simulink model "flight_model"  (Simulink 7.6)
settings: Solver=ode23  StartTime=0.0  StopTime=30  RelTol=1e-3
values from neighbouring files (symbols this model uses):
  initial_pos = [[44.98 -76.96] * pi / 180 0]    [Geo_model_sim.m]
  Uo = trim_values(10:13)    [Geo_Find_Trim.m]
  Xo = trim_values(1:9)    [Geo_Find_Trim.m]
undefined symbols (not defined in the file or in its folder): aerosimlib, Earth, WGS
settings Model: Creator=gblouin  LastModifiedBy=aholtzma
settings DataIOCC: ExternalInput=[u]  LimitDataPoints=off  SaveOutput=off  SignalLogging=off  DSMLogging=off  OutputSaveName=xout
settings OptimizationCC: InlineParams=on  InlineInvariantSignals=on  EfficientFloat2IntCast=on
settings DebuggingCC: SaveWithParameterizedLinksMsg=none  MultiTaskDSMMsg=warning  MultiTaskCondExecSysMsg=none  StrictBusMsg=Warning
settings SFSimCC: SimParseCustomCode=off
settings RTWCC: IncludeERTFirstTime=on
settings GRTTargetCC: TargetFcnLib=ansi_tfl_tmw.mat

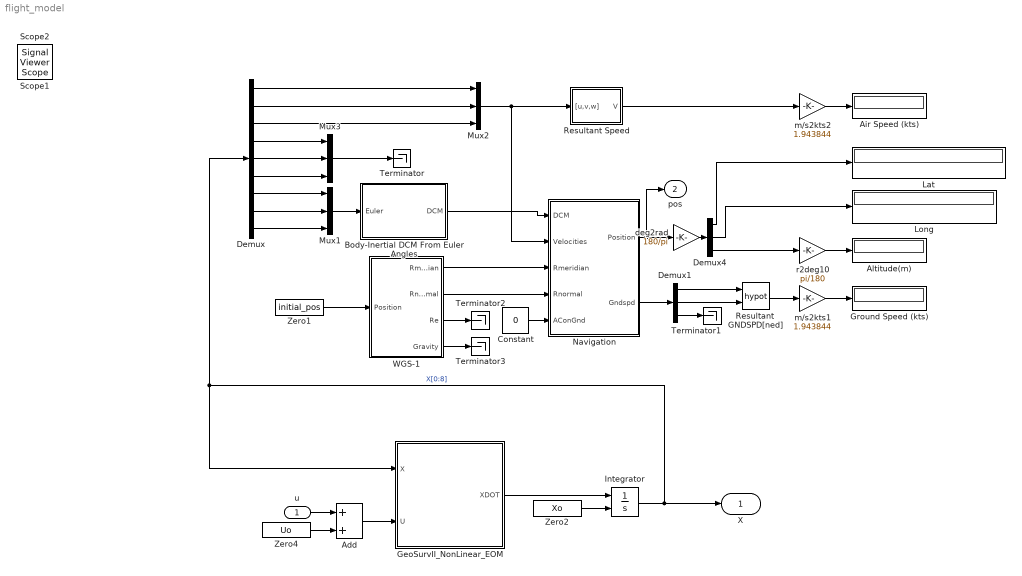
== system flight_model ==
  u : Inport  PortDimensions=4
  Add : Sum
  Air Speed (kts) : Display
  Altitude(m) : Display
  Body-Inertial DCM From Euler Angles : Subsystem  AncestorBlock=aerosimlib/Transformations/Body-Inertial DCM From Euler Angles
  Constant : Constant  Value=0
  Demux : Demux  Outputs=9
  Demux1 : Demux  Outputs=3
  Demux4 : Demux  Outputs=3
  GeoSurvII_NonLinear_EOM : Stateflow chart  TreatAsAtomicUnit=on
  Ground Speed (kts) : Display
  Integrator : Integrator  InitialConditionSource=external  InitialCondition=Xo
  Lat : Display
  Long : Display
  Mux1 : Mux  Inputs=3
  Mux2 : Mux  Inputs=3
  Mux3 : Mux  Inputs=3
  Navigation : Subsystem
  Resultant  GNDSPD[ned] : Math  Operator=hypot  SaturateOnIntegerOverflow=on
  Resultant Speed : Subsystem  AncestorBlock=aerosimlib/Equations of Motion/Body-Frame EOM/Kinematics (Euler)
  Terminator{,1..3} (4 alike) : Terminator
  WGS-1 : Subsystem  AncestorBlock=aerosimlib/Earth/WGS-84
  Zero1 : Constant  Value=initial_pos
  Zero2 : Constant  Value=Xo
  Zero4 : Constant  Value=Uo
  deg2rad : Gain  Gain=180/pi
  m/s2kts1 : Gain  Gain=1.943844
  m/s2kts2 : Gain  Gain=1.943844
  r2deg10 : Gain  Gain=pi/180
  X : Outport
  pos : Outport  Port=2
  Scope1 : SignalViewerScope  IOType=viewer  NumInputPorts=2  ZoomMode=xonly  RefreshTime=1.500000
      settings: TimeRange=100  YMin=-3.5~-2.84987e-012  YMax=0.5~-2.57845e-012  MaxDataPoints=20000
  Scope2 : SignalViewerScope  IOType=viewer  NumInputPorts=2  ZoomMode=xonly  RefreshTime=1.500000
      settings: TimeRange=100  YMin=-40~9.16954  YMax=10~10.1348  MaxDataPoints=20000
  wires:
  Navigation/1(Position) -> deg2rad/1, pos/1
  Demux4/1 -> Lat/1
  Demux4/2 -> Long/1
  deg2rad/1 -> Demux4/1
  Demux4/3 -> r2deg10/1
  r2deg10/1 -> Altitude(m)/1
  Navigation/2(Gndspd) -> Demux1/1
  Demux1/1 -> Resultant  GNDSPD[ned]/1
  Demux1/2 -> Resultant  GNDSPD[ned]/2
  Integrator/1 -> GeoSurvII_NonLinear_EOM/1(X), Demux/1, X/1  "X[0:8]"
  Zero2/1 -> Integrator/2
  GeoSurvII_NonLinear_EOM/1(XDOT) -> Integrator/1
  Demux/1 -> Mux2/1
  Resultant  GNDSPD[ned]/1 -> m/s2kts1/1
  m/s2kts1/1 -> Ground Speed (kts)/1
  WGS-1/1(Rmeridian) -> Navigation/3(Rmeridian)
  WGS-1/2(Rnormal) -> Navigation/4(Rnormal)
  Body-Inertial DCM From Euler Angles/1(DCM) -> Navigation/1(DCM)
  Mux2/1 -> Navigation/2(Velocities), Resultant Speed/1("[u,v,w]")
  Zero1/1 -> WGS-1/1(Position)
  Resultant Speed/1(V) -> m/s2kts2/1
  m/s2kts2/1 -> Air Speed (kts)/1
  Demux/2 -> Mux2/2
  Demux/3 -> Mux2/3
  Demux/7 -> Mux1/1
  Demux/8 -> Mux1/2
  Demux/9 -> Mux1/3
  Mux1/1 -> Body-Inertial DCM From Euler Angles/1(Euler)
  Demux/4 -> Mux3/1
  Demux/5 -> Mux3/2
  Demux/6 -> Mux3/3
  Add/1 -> GeoSurvII_NonLinear_EOM/2(U)
  u/1 -> Add/1
  Zero4/1 -> Add/2
  Mux3/1 -> Terminator/1
  Demux1/3 -> Terminator1/1
  WGS-1/3(Re) -> Terminator2/1
  WGS-1/4(Gravity) -> Terminator3/1
  Constant/1 -> Navigation/5(AConGnd)

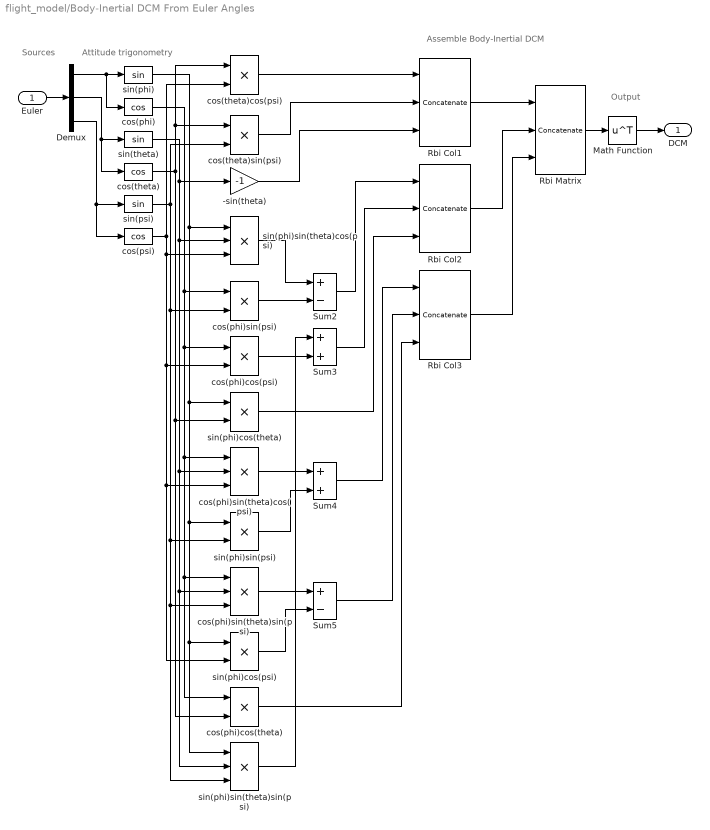
== system flight_model/Body-Inertial DCM From Euler Angles ==
  note: Sources
  note: Assemble Body-Inertial DCM
  note: Output
  note: Attitude trigonometry
  Euler : Inport  PortDimensions=[3 1]
  -sin(theta) : Gain  Gain=-1  SaturateOnIntegerOverflow=on  OutDataTypeStr=Inherit: Same as input  ParamDataTypeStr=Inherit: Same as input
  Demux : Demux  Outputs=3
  Math Function : Math  Operator=transpose  SaturateOnIntegerOverflow=on
  Rbi Matrix : Concatenate  NumInputs=3  Mode=Multidimensional array  ConcatenateDimension=2
  Rbi Col1 : Concatenate  NumInputs=3  Mode=Multidimensional array
  Rbi Col2 : Concatenate  NumInputs=3  Mode=Multidimensional array
  Rbi Col3 : Concatenate  NumInputs=3  Mode=Multidimensional array
  Sum2 : Sum  Inputs=+-  SaturateOnIntegerOverflow=on  InputSameDT=on  OutDataTypeStr=Inherit: Same as first input
  Sum3 : Sum  SaturateOnIntegerOverflow=on  InputSameDT=on  OutDataTypeStr=Inherit: Same as first input
  Sum4 : Sum  SaturateOnIntegerOverflow=on  InputSameDT=on  OutDataTypeStr=Inherit: Same as first input
  Sum5 : Sum  Inputs=+-  SaturateOnIntegerOverflow=on  InputSameDT=on  OutDataTypeStr=Inherit: Same as first input
  cos(phi) : Trigonometry  Operator=cos
  cos(phi)cos(psi) : Product  SaturateOnIntegerOverflow=on  InputSameDT=on  OutDataTypeStr=Inherit: Same as first input
  cos(phi)cos(theta) : Product  SaturateOnIntegerOverflow=on  InputSameDT=on  OutDataTypeStr=Inherit: Same as first input
  cos(phi)sin(psi) : Product  SaturateOnIntegerOverflow=on  InputSameDT=on  OutDataTypeStr=Inherit: Same as first input
  cos(phi)sin(theta)cos(psi) : Product  Inputs=3  SaturateOnIntegerOverflow=on  InputSameDT=on  OutDataTypeStr=Inherit: Same as first input
  cos(phi)sin(theta)sin(psi) : Product  Inputs=3  SaturateOnIntegerOverflow=on  InputSameDT=on  OutDataTypeStr=Inherit: Same as first input
  cos(psi) : Trigonometry  Operator=cos
  cos(theta) : Trigonometry  Operator=cos
  cos(theta)cos(psi) : Product  SaturateOnIntegerOverflow=on  InputSameDT=on  OutDataTypeStr=Inherit: Same as first input
  cos(theta)sin(psi) : Product  SaturateOnIntegerOverflow=on  InputSameDT=on  OutDataTypeStr=Inherit: Same as first input
  sin(phi) : Trigonometry
  sin(phi)cos(psi) : Product  SaturateOnIntegerOverflow=on  InputSameDT=on  OutDataTypeStr=Inherit: Same as first input
  sin(phi)cos(theta) : Product  SaturateOnIntegerOverflow=on  InputSameDT=on  OutDataTypeStr=Inherit: Same as first input
  sin(phi)sin(psi) : Product  SaturateOnIntegerOverflow=on  InputSameDT=on  OutDataTypeStr=Inherit: Same as first input
  sin(phi)sin(theta)cos(psi) : Product  Inputs=3  SaturateOnIntegerOverflow=on  InputSameDT=on  OutDataTypeStr=Inherit: Same as first input
  sin(phi)sin(theta)sin(psi) : Product  Inputs=3  SaturateOnIntegerOverflow=on  InputSameDT=on  OutDataTypeStr=Inherit: Same as first input
  sin(psi) : Trigonometry
  sin(theta) : Trigonometry
  DCM : Outport
  wires:
  Euler/1 -> Demux/1
  Rbi Col1/1 -> Rbi Matrix/1
  Rbi Col2/1 -> Rbi Matrix/2
  Rbi Col3/1 -> Rbi Matrix/3
  Rbi Matrix/1 -> Math Function/1
  Demux/1 -> sin(phi)/1, cos(phi)/1
  Demux/2 -> cos(theta)/1, sin(theta)/1
  Demux/3 -> cos(psi)/1, sin(psi)/1
  sin(phi)/1 -> sin(phi)sin(psi)/1, sin(phi)cos(psi)/1, sin(phi)sin(theta)sin(psi)/1, sin(phi)cos(theta)/1, sin(phi)sin(theta)cos(psi)/1
  cos(phi)/1 -> cos(phi)cos(theta)/1, cos(phi)sin(theta)sin(psi)/1, cos(phi)sin(theta)cos(psi)/1, cos(phi)cos(psi)/1, cos(phi)sin(psi)/1
  sin(theta)/1 -> cos(phi)sin(theta)cos(psi)/2, cos(phi)sin(theta)sin(psi)/2, sin(phi)sin(theta)sin(psi)/2, sin(phi)sin(theta)cos(psi)/2, -sin(theta)/1
  cos(theta)/1 -> cos(phi)cos(theta)/2, sin(phi)cos(theta)/2, cos(theta)sin(psi)/1, cos(theta)cos(psi)/1
  sin(psi)/1 -> sin(phi)sin(psi)/2, cos(phi)sin(theta)sin(psi)/3, sin(phi)sin(theta)sin(psi)/3, cos(phi)sin(psi)/2, cos(theta)sin(psi)/2
  cos(psi)/1 -> sin(phi)cos(psi)/2, cos(phi)sin(theta)cos(psi)/3, cos(phi)cos(psi)/2, sin(phi)sin(theta)cos(psi)/3, cos(theta)cos(psi)/2
  cos(phi)sin(psi)/1 -> Sum2/2
  cos(phi)cos(psi)/1 -> Sum3/2
  sin(phi)sin(theta)cos(psi)/1 -> Sum2/1
  cos(phi)sin(theta)cos(psi)/1 -> Sum4/1
  sin(phi)sin(psi)/1 -> Sum4/2
  cos(phi)sin(theta)sin(psi)/1 -> Sum5/1
  sin(phi)cos(psi)/1 -> Sum5/2
  cos(theta)cos(psi)/1 -> Rbi Col1/1
  cos(theta)sin(psi)/1 -> Rbi Col1/2
  -sin(theta)/1 -> Rbi Col1/3
  Sum2/1 -> Rbi Col2/1
  Sum3/1 -> Rbi Col2/2
  sin(phi)cos(theta)/1 -> Rbi Col2/3
  Sum4/1 -> Rbi Col3/1
  Sum5/1 -> Rbi Col3/2
  cos(phi)cos(theta)/1 -> Rbi Col3/3
  Math Function/1 -> DCM/1
  sin(phi)sin(theta)sin(psi)/1 -> Sum3/1

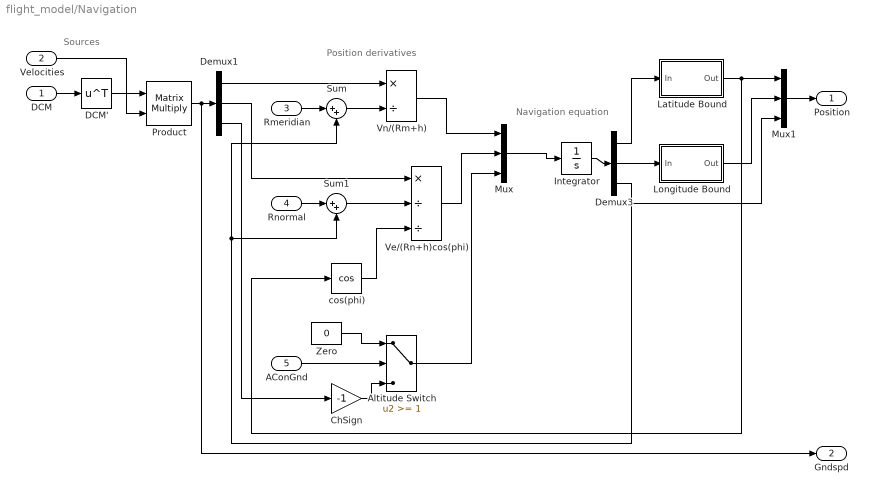
== system flight_model/Navigation ==
  note: Navigation equation
  note: Position derivatives
  note: Sources
  DCM : Inport  PortDimensions=[3 3]
  Velocities : Inport  Port=2  PortDimensions=[3 1]
  Rmeridian : Inport  Port=3  PortDimensions=1
  Rnormal : Inport  Port=4  PortDimensions=1
  AConGnd : Inport  Port=5  PortDimensions=1
  Altitude Switch : Switch  Threshold=1  SaturateOnIntegerOverflow=on  InputSameDT=on
  ChSign : Gain  Gain=-1  SaturateOnIntegerOverflow=on  OutDataTypeStr=Inherit: Same as input  ParamDataTypeStr=Inherit: Same as input
  DCM' : Math  Operator=transpose  SaturateOnIntegerOverflow=on
  Demux1 : Demux  Outputs=3
  Demux3 : Demux  Outputs=3
  Integrator : Integrator  InitialCondition=[41.684028*pi/180 -81.389750*pi/180 500]
  Latitude Bound : Subsystem
      mask Type: Latitude bound
      mask Description: Bounds the latitude to [-pi/2, pi/2]. When the lower bound is exceeded the latitude is increasing again; when the upper bound is exceeded the latitude is decreasing.
  Longitude Bound : Subsystem
      mask Type: Longitude bound
      mask Description: Bounds the longitude to [-pi, pi]. When -pi bound is exceeded the longitude wraps back to pi; when the pi bound is exceeded the longitude wraps back to -pi.
  Mux : Mux  Inputs=3
  Mux1 : Mux  Inputs=3
  Product : Product  Multiplication=Matrix(*)  SaturateOnIntegerOverflow=on  InputSameDT=on  OutDataTypeStr=Inherit: Same as first input
  Sum : Sum  Inputs=|++  SaturateOnIntegerOverflow=on  InputSameDT=on  OutDataTypeStr=Inherit: Same as first input
  Sum1 : Sum  Inputs=|++  SaturateOnIntegerOverflow=on  InputSameDT=on  OutDataTypeStr=Inherit: Same as first input
  Ve/(Rn+h)cos(phi) : Product  Inputs=*//  SaturateOnIntegerOverflow=on  InputSameDT=on  OutDataTypeStr=Inherit: Same as first input
  Vn/(Rm+h) : Product  Inputs=*/  SaturateOnIntegerOverflow=on  InputSameDT=on  OutDataTypeStr=Inherit: Same as first input
  Zero : Constant  Value=0
  cos(phi) : Trigonometry  Operator=cos
  Position : Outport
  Gndspd : Outport  Port=2
  wires:
  Latitude Bound/1(Out) -> Mux1/1, cos(phi)/1
  Mux1/1 -> Position/1
  Longitude Bound/1(Out) -> Mux1/2
  Demux3/1 -> Latitude Bound/1(In)
  Demux3/2 -> Longitude Bound/1(In)
  Demux3/3 -> Mux1/3, Sum1/2, Sum/2
  cos(phi)/1 -> Ve/(Rn+h)cos(phi)/3
  Integrator/1 -> Demux3/1
  Mux/1 -> Integrator/1
  Altitude Switch/1 -> Mux/3
  ChSign/1 -> Altitude Switch/3
  Zero/1 -> Altitude Switch/1
  AConGnd/1 -> Altitude Switch/2
  DCM'/1 -> Product/1
  DCM/1 -> DCM'/1
  Ve/(Rn+h)cos(phi)/1 -> Mux/2
  Sum1/1 -> Ve/(Rn+h)cos(phi)/2
  Vn/(Rm+h)/1 -> Mux/1
  Sum/1 -> Vn/(Rm+h)/2
  Rnormal/1 -> Sum1/1
  Rmeridian/1 -> Sum/1
  Product/1 -> Gndspd/1, Demux1/1
  Demux1/2 -> Ve/(Rn+h)cos(phi)/1
  Demux1/3 -> ChSign/1
  Demux1/1 -> Vn/(Rm+h)/1
  Velocities/1 -> Product/2

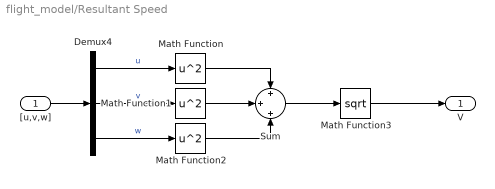
== system flight_model/Resultant Speed ==
  "[u,v,w]" : Inport  PortDimensions=[3 1]
  Demux4 : Demux  Outputs=3
  Math Function : Math  Operator=square  SaturateOnIntegerOverflow=on
  Math Function1 : Math  Operator=square  SaturateOnIntegerOverflow=on
  Math Function2 : Math  Operator=square  SaturateOnIntegerOverflow=on
  Math Function3 : Math  Operator=sqrt  SaturateOnIntegerOverflow=on
  Sum : Sum  Inputs=+|+|+
  V : Outport
  wires:
  Demux4/2 -> Math Function1/1  "v"
  Demux4/3 -> Math Function2/1  "w"
  Math Function/1 -> Sum/1
  Math Function1/1 -> Sum/2
  Math Function2/1 -> Sum/3
  Sum/1 -> Math Function3/1
  Math Function3/1 -> V/1
  Demux4/1 -> Math Function/1  "u"
  "[u,v,w]"/1 -> Demux4/1

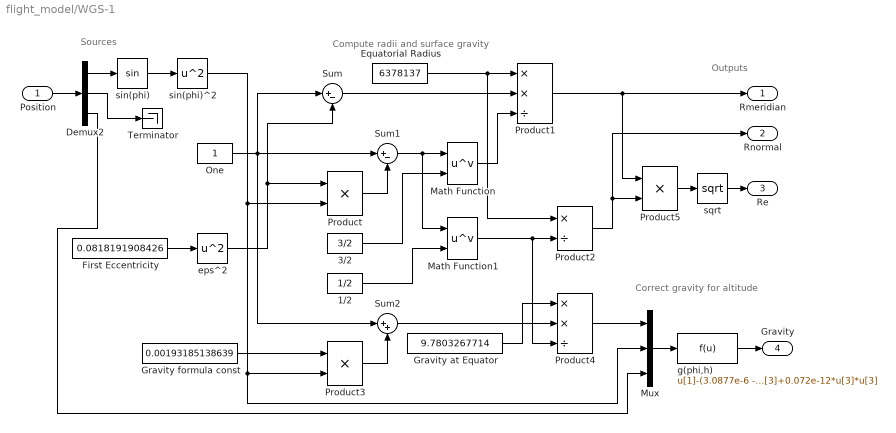
== system flight_model/WGS-1 ==
  note: Sources
  note: Compute radii and surface gravity
  note: Correct gravity for altitude
  note: Outputs
  Position : Inport
  1/2 : Constant  Value=1/2
  3/2 : Constant  Value=3/2
  Demux2 : Demux  Outputs=3
  Equatorial Radius : Constant  Value=6378137
  First Eccentricity : Constant  Value=0.0818191908426
  Gravity at Equator : Constant  Value=9.7803267714
  Gravity formula const : Constant  Value=0.00193185138639
  Math Function : Math  Operator=pow  SaturateOnIntegerOverflow=on
  Math Function1 : Math  Operator=pow  SaturateOnIntegerOverflow=on
  Mux : Mux  Inputs=3
  One : Constant
  Product : Product  SaturateOnIntegerOverflow=on  InputSameDT=on  OutDataTypeStr=Inherit: Same as first input
  Product1 : Product  Inputs=**/  SaturateOnIntegerOverflow=on  InputSameDT=on  OutDataTypeStr=Inherit: Same as first input
  Product2 : Product  Inputs=*/  SaturateOnIntegerOverflow=on  InputSameDT=on  OutDataTypeStr=Inherit: Same as first input
  Product3 : Product  SaturateOnIntegerOverflow=on  InputSameDT=on  OutDataTypeStr=Inherit: Same as first input
  Product4 : Product  Inputs=**/  SaturateOnIntegerOverflow=on  InputSameDT=on  OutDataTypeStr=Inherit: Same as first input
  Product5 : Product  SaturateOnIntegerOverflow=on  InputSameDT=on  OutDataTypeStr=Inherit: Same as first input
  Sum : Sum  Inputs=|+-  SaturateOnIntegerOverflow=on  InputSameDT=on  OutDataTypeStr=Inherit: Same as first input
  Sum1 : Sum  Inputs=|+-  SaturateOnIntegerOverflow=on  InputSameDT=on  OutDataTypeStr=Inherit: Same as first input
  Sum2 : Sum  Inputs=|++  SaturateOnIntegerOverflow=on  InputSameDT=on  OutDataTypeStr=Inherit: Same as first input
  Terminator : Terminator
  eps^2 : Math  Operator=square  SaturateOnIntegerOverflow=on
  g(phi,h) : Fcn  Expr=u[1]-(3.0877e-6 - 0.0044e-6*u[2])*u[3]+0.072e-12*u[3]*u[3]
  sin(phi) : Trigonometry
  sin(phi)^2 : Math  Operator=square  SaturateOnIntegerOverflow=on
  sqrt : Math  Operator=sqrt  SaturateOnIntegerOverflow=on
  Rmeridian : Outport
  Rnormal : Outport  Port=2
  Re : Outport  Port=3
  Gravity : Outport  Port=4
  wires:
  sqrt/1 -> Re/1
  Product5/1 -> sqrt/1
  First Eccentricity/1 -> eps^2/1
  eps^2/1 -> Sum/2, Product/1
  sin(phi)/1 -> sin(phi)^2/1
  sin(phi)^2/1 -> Product/2, Product3/2, Mux/2
  One/1 -> Sum1/1, Sum2/1, Sum/1
  Product/1 -> Sum1/2
  Sum1/1 -> Math Function/1, Math Function1/1
  3/2/1 -> Math Function/2
  1/2/1 -> Math Function1/2
  Equatorial Radius/1 -> Product1/1, Product2/1
  Sum/1 -> Product1/2
  Math Function/1 -> Product1/3
  Math Function1/1 -> Product2/2, Product4/3
  Product1/1 -> Rmeridian/1, Product5/1
  Product2/1 -> Rnormal/1, Product5/2
  Gravity formula const/1 -> Product3/1
  Product3/1 -> Sum2/2
  Gravity at Equator/1 -> Product4/1
  Sum2/1 -> Product4/2
  Product4/1 -> Mux/1
  Position/1 -> Demux2/1
  Demux2/1 -> sin(phi)/1
  Demux2/2 -> Terminator/1
  Mux/1 -> g(phi,h)/1
  g(phi,h)/1 -> Gravity/1
  Demux2/3 -> Mux/3

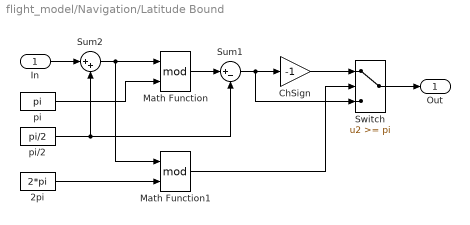
== system flight_model/Navigation/Latitude Bound ==
  In : Inport
  2pi : Constant  Value=2*pi
  ChSign : Gain  Gain=-1  SaturateOnIntegerOverflow=on  OutDataTypeStr=Inherit: Same as input  ParamDataTypeStr=Inherit: Same as input
  Math Function : Math  Operator=mod  SaturateOnIntegerOverflow=on
  Math Function1 : Math  Operator=mod  SaturateOnIntegerOverflow=on
  Sum1 : Sum  Inputs=|+-  SaturateOnIntegerOverflow=on  InputSameDT=on  OutDataTypeStr=Inherit: Same as first input
  Sum2 : Sum  Inputs=|++  SaturateOnIntegerOverflow=on  InputSameDT=on  OutDataTypeStr=Inherit: Same as first input
  Switch : Switch  Threshold=pi  SaturateOnIntegerOverflow=on  InputSameDT=on
  pi : Constant  Value=pi
  pi/2 : Constant  Value=pi/2
  Out : Outport
  wires:
  2pi/1 -> Math Function1/2
  ChSign/1 -> Switch/1
  Sum2/1 -> Math Function1/1, Math Function/1
  In/1 -> Sum2/1
  Switch/1 -> Out/1
  Math Function1/1 -> Switch/2
  Sum1/1 -> Switch/3, ChSign/1
  pi/2/1 -> Sum2/2, Sum1/2
  Math Function/1 -> Sum1/1
  pi/1 -> Math Function/2

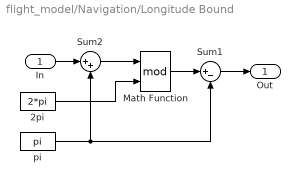
== system flight_model/Navigation/Longitude Bound ==
  In : Inport
  2pi : Constant  Value=2*pi
  Math Function : Math  Operator=mod  SaturateOnIntegerOverflow=on
  Sum1 : Sum  Inputs=|+-  SaturateOnIntegerOverflow=on  InputSameDT=on  OutDataTypeStr=Inherit: Same as first input
  Sum2 : Sum  Inputs=|++  SaturateOnIntegerOverflow=on  InputSameDT=on  OutDataTypeStr=Inherit: Same as first input
  pi : Constant  Value=pi
  Out : Outport
  wires:
  Math Function/1 -> Sum1/1
  2pi/1 -> Math Function/2
  In/1 -> Sum2/1
  Sum2/1 -> Math Function/1
  pi/1 -> Sum2/2, Sum1/2
  Sum1/1 -> Out/1

== matlab function GeoSurvII_NonLinear_EOM ==
  settings: fimath=|
      | fimath(...
      | 'RoundMode', 'floor',...
      | 'OverflowMode', 'wrap',...
      | 'ProductMode', 'KeepLSB', 'ProductWordLength', 32,...
      | 'SumMode', 'KeepLSB', 'SumWordLength', 32,...
      | 'CastBeforeSum', false)
  data: X input double; XDOT output double; U input double
function XDOT = Geo_model(X,U)

%GEO_MODEL Full 6 DOF model for GeoSurv II aircraft
%
%   [XDOT] = GEO_MODEL(X,U) returns the state derivatives, XDOT, given the
%   current state and inputs, X and U.  The constants are the nominal
%   constants.
%
%   State vector X and input vector U is defined as
%   
%       X = [u;v;w;p;q;r;phi;theta;psi] = [x1;x2;x3;x4;x5;x6;x7;x8;x9]
%       U = [d_A;d_E;d_R;d_th] = [u1;u2;u3;u4]
%
%
%Created by Christopher Lum
%lum@u.washington.edu
%Modified for GeoSurv II aircraft by Guillaume Blouin


%-----------------------CONSTANTS-------------------------------
%Unit conversions
lb_to_kg = 0.45359237;          %Unit conversion (pounds to kilograms)
in_to_m = 0.0254;               %Unit conversion (inches to meters)
ft_to_m = 0.3048;               %Unit conversion (feet to meters)
kt_to_ms = 0.514444;            %Unit conversion (knots to meters/second)
slug_to_kg = 14.593903;         %Unit conversion (slugs to kilograms)

%Mass moments of inertia
Ixx = 25.2589*slug_to_kg*ft_to_m^2;
Iyy = 32.8379*slug_to_kg*ft_to_m^2;
Izz = 47.0740*slug_to_kg*ft_to_m^2;
Ixz = 0*slug_to_kg*ft_to_m^2;

%Nominal vehicle constants (problem 1)
m = 186*lb_to_kg;               %Aircraft total mass (kg)
cbar = 27*in_to_m;              %Mean Aerodynamic Chord (m)
lt = 108.55*in_to_m;            %Distance by AC of tail and body (m)
S = 36*ft_to_m^2;               %Wing planform area (m^2)
St = 9.5*ft_to_m^2;             %Tail planform area (m^2)
i = -2*pi/180;                  %Tail incidence angle (rad)
AR = 7.11;                      %Aspect ratio
e = 0.836;                      %Oswalt's efficiency factor

Xcg = 0.25*cbar;                %x position of CoG in Fm (m)
Ycg = 0;                        %y position of CoG in Fm (m)
Zcg = 0.037*cbar;               %z position of CoG in Fm (m)

%Engine inputs
Xapt = 0;                       %x position of engine force in Fm (m)
Yapt = 0;                       %y position of engine force in Fm (m)
Zapt = 0.1405;                  %z position of engine force in Fm (m)

%Other constants
rho = 1.225;                    %Air density (kg/m^3)
g = 9.81;                       %Gravitational acceleration (m/s^2)
depsda = 0.33;                  %Change in downwash w.r.t. alpha (rad/rad)
alpha_L0 = -4*pi/180;           %Zero lift angle of attack (rad)

%Stability Derivatives (output from Justin Koning's Linear Model)
CXu = -0.096;
CXa = 0.19042;
CXadot = 0;
CXq = 0;
CXde = 0;
 
CZu = -1.0381;
CZa = -5.9345;
CZadot = -1.1763;
CZq = -5.6462;
CZde = -0.15543;
 
Cmu = 0;
Cma = -0.6094;
Cmadot = -4.496;
Cmq = -14.9865;
Cmde = -0.5958;
 
CYb = -0.5291;
CYbdot = 0;
CYp = 0.029801;
CYr = 0.4479;
CYda = 0;
CYdr = 0.13127;
 
Clb = -0.033192;
Clp = -0.49901;
Clr = 0.14677;
Clda = 0.14359;
Cldr = 0.0035059;
 
Cnb = 0.20878;
Cnbdot = 0;
Cnp = -0.071083;
Cnr = -0.20574;
Cnda = -0.0051955;
Cndr = -0.070618;

%Convert CZ to CL
CLu = -CZu;
CLa = -CZa;
CLadot = -CZadot;
CLq = -CZq;
CLde = -CZde;

%Other Stability Derivatives (from AERO database)
CDo = 0.0222;
CMo = -0.1003;
CLa_t = 3.544;


%--------------------------STATE VECTOR----------------------------------
%Extract state vector
x1 = X(1);                              %u
x2 = X(2);                              %v
x3 = X(3);                              %w
x4 = X(4);                              %p
x5 = X(5);                              %q
x6 = X(6);                              %r
x7 = X(7);                              %phi
x8 = X(8);                              %theta
x9 = X(9);                              %psi

u1 = U(1);                              %d_A (aileron)
u2 = U(2);                              %d_E (elevator)
u3 = U(3);                              %d_R (rudder)
u4 = U(4);                              %d_th (throttle)


%---------------INTERMEDIATE VARIABLES------------------------
%Calculate airspeed
Va = sqrt(x1^2 + x2^2 + x3^2);

%Calculate alpha and beta
alpha = atan(x3/x1);
beta = asin(x2/Va);

%Calculate dynamic pressure
Q = 0.5*rho*Va^2;

%Also define the vectors wbe_b and V_b 
wbe_b = [x4;x5;x6];
V_b = [x1;x2;x3];


%---------------AERODYNAMIC FORCE COEFFICIENTS----------------
%Calculate the CL_wb
if Va<(35.6*kt_to_ms)
end

if alpha<= 17*pi*180
    CL_wb=CLa*(alpha-alpha_L0);
elseif alpha>17*pi*180
    CL_wb=-5*10^-5*alpha^4+0.0034*alpha^3-0.092*alpha^2+1.1374*alpha-4.2971;
else
    CL_wb=2.75;
end

%Calculate CL_t
epsilon = depsda*(alpha - alpha_L0);
alpha_t = alpha - epsilon + i + CLq*x5*lt/Va;
CL_t = CLa_t*alpha_t + CLde*u2;

%Total lift force
CL = CL_wb + CL_t*(St/S);

%Total drag force (neglecting tail)
CD = CDo + CL^2/(pi*AR*e);

%Calculate sideforce
CY = CYb*beta + CYdr*u3 + CYr*x6;


%--------------DIMENSIONAL AERODYNAMIC FORCES---------------------
%Calculate the actual dimensional forces.  These are in F_s (stability axis)
FA_s = [-CD*Q*S;
         CY*Q*S;
        -CL*Q*S];
    
%Rotate these forces to F_b (body axis)
C_bs = [cos(alpha) 0 -sin(alpha);
        0 1 0;
        sin(alpha) 0 cos(alpha)];
    
FA_b = C_bs*FA_s;


%-------------AERODYNAMIC MOMENT COEFFICIENTS---------------
%Calculate the moments in Fb.  Define eta, dCMdx and dCMdu
eta11 = Clb*beta;
eta21 = CMo - (CLa_t*(St*lt)/(S*cbar))*(alpha - epsilon);
eta31 = Cnb*beta;

eta = [eta11;
       eta21;
       eta31];

dCMdx = (cbar/Va)*[Clp 0 Clr;
                    0 (Cmq*(St*lt^2)/(S*cbar^2)) 0;
                    Cnp 0 Cnr];
              
dCMdu = [Clda 0 Cldr;
          0 (-CLa_t*(St*lt)/(S*cbar)) 0;
          0 0 Cndr];

%Now calculate CM = [Cl;Cm;Cn] about Aerodynamic center in Fb
CMac_b = eta + dCMdx*wbe_b + dCMdu*[u1;u2;u3];

%Transfer now to CoG.
CX = -CD*cos(alpha) + CL*sin(alpha);
CZ = -CL*cos(alpha) - CD*sin(alpha);

A = (1/cbar)*[0 CZ -CY;
              -CZ 0 CX;
              CY -CX 0];

zeta = [(Xcg-0.12*cbar);
        -Ycg;
        Zcg];

CMcg_b = CMac_b + A*zeta;


%---------------DIMENSIONAL AERODYNAMIC MOMENTS---------------------
%Calculate the dimensional moments in Fb about cg
MAcg_b = CMcg_b*(Q*S*cbar);


%-----------------ENGINE FORCE & MOMENT----------------------------
%Now effect of engine.  First, calculate the thrust of engine
F = u4*m*g;

%Assuming that engine thrust is aligned with Fb, we have
FE_b = [F;0;0];
  
%Now engine moment due to offset of engine thrust from CoG.
mew = [Xcg - Xapt;
        Yapt - Ycg;
        Zcg - Zapt];


MEcg_b = cross(mew,FE_b);


%--------------------GRAVITY EFFECTS--------------------------------
%Calculate gravitational forces in the body frame.  This causes no moment
%about CoG.
g_b = [-g*sin(x8);
        g*cos(x8)*sin(x7);
        g*cos(x8)*cos(x7)];
  
Fg_b = m*g_b;


%-------------------STATE DERIVATIVES------------------------------
%Inertia matrix
Ib = m*[Ixx 0 Ixz;
        0 Iyy 0;
        Ixz 0 Izz];
    
%Inverse of inertia matrix 
invIb = inv(Ib);

%Form F_b (all the forces in Fb) and calculate udot, vdot, wdot
F_b = Fg_b + FE_b + FA_b;
x1to3dot = (1/m)*F_b - cross(wbe_b,V_b);

%Form Mcg_b (all moments about CoG in Fb) and calculate pdot, qdot, rdot.
Mcg_b = MAcg_b + MEcg_b;
x4to6dot = invIb*(Mcg_b - cross(wbe_b,Ib*wbe_b));

%Calculate phidot,thetadot, and psidot    
H_phi = [1 sin(x7)*tan(x8) cos(x7)*tan(x8);
         0 cos(x7) -sin(x7);
         0 sin(x7)/cos(x8) cos(x7)/cos(x8)];
    
x7to9dot = H_phi*wbe_b;

%Place in first order form
XDOT = [x1to3dot(1);                    %udot
        x1to3dot(2);                    %vdot
        x1to3dot(3);                    %wdot
        x4to6dot(1);                    %pdot
        x4to6dot(2);                    %qdot
        x4to6dot(3);                    %rdot
        x7to9dot(1);                    %phidot
        x7to9dot(2);                    %thetadot
        x7to9dot(3)];                   %psidot
